simulink model "pokus07_video"  (R2023a)
settings: Solver=VariableStepAuto  StartTime=0.0  StopTime=10.0  RelTol=1e-3
undefined symbols (not defined in the file): c
libraries: Miscellaneous x840, Memory_Blocks_Lib x251, Decoders_Lib x10, simulink_extras x10, Counters_Lib x4, Bit_Multiplexers_Lib x1, Byte_Multiplexers_Lib x1
(part 4 of 5)

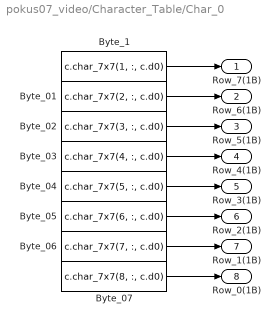
== system pokus07_video/Character_Table/Char_0 ==
  Byte_01 : Constant  Value=c.char_7x7(2, :, c.d0)  OutDataTypeStr=uint8
  Byte_02 : Constant  Value=c.char_7x7(3, :, c.d0)  OutDataTypeStr=uint8
  Byte_03 : Constant  Value=c.char_7x7(4, :, c.d0)  OutDataTypeStr=uint8
  Byte_04 : Constant  Value=c.char_7x7(5, :, c.d0)  OutDataTypeStr=uint8
  Byte_05 : Constant  Value=c.char_7x7(6, :, c.d0)  OutDataTypeStr=uint8
  Byte_06 : Constant  Value=c.char_7x7(7, :, c.d0)  OutDataTypeStr=uint8
  Byte_07 : Constant  Value=c.char_7x7(8, :, c.d0)  OutDataTypeStr=uint8
  Byte_1 : Constant  Value=c.char_7x7(1, :, c.d0)  OutDataTypeStr=uint8
  Row_7(1B) : Outport
  Row_6(1B) : Outport  Port=2
  Row_5(1B) : Outport  Port=3
  Row_4(1B) : Outport  Port=4
  Row_3(1B) : Outport  Port=5
  Row_2(1B) : Outport  Port=6
  Row_1(1B) : Outport  Port=7
  Row_0(1B) : Outport  Port=8
  wires:
  Byte_06/1 -> Row_1(1B)/1
  Byte_05/1 -> Row_2(1B)/1
  Byte_04/1 -> Row_3(1B)/1
  Byte_07/1 -> Row_0(1B)/1
  Byte_01/1 -> Row_6(1B)/1
  Byte_02/1 -> Row_5(1B)/1
  Byte_1/1 -> Row_7(1B)/1
  Byte_03/1 -> Row_4(1B)/1

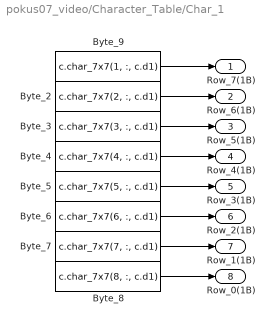
== system pokus07_video/Character_Table/Char_1 ==
  Byte_2 : Constant  Value=c.char_7x7(2, :, c.d1)  OutDataTypeStr=uint8
  Byte_3 : Constant  Value=c.char_7x7(3, :, c.d1)  OutDataTypeStr=uint8
  Byte_4 : Constant  Value=c.char_7x7(4, :, c.d1)  OutDataTypeStr=uint8
  Byte_5 : Constant  Value=c.char_7x7(5, :, c.d1)  OutDataTypeStr=uint8
  Byte_6 : Constant  Value=c.char_7x7(6, :, c.d1)  OutDataTypeStr=uint8
  Byte_7 : Constant  Value=c.char_7x7(7, :, c.d1)  OutDataTypeStr=uint8
  Byte_8 : Constant  Value=c.char_7x7(8, :, c.d1)  OutDataTypeStr=uint8
  Byte_9 : Constant  Value=c.char_7x7(1, :, c.d1)  OutDataTypeStr=uint8
  Row_7(1B) : Outport
  Row_6(1B) : Outport  Port=2
  Row_5(1B) : Outport  Port=3
  Row_4(1B) : Outport  Port=4
  Row_3(1B) : Outport  Port=5
  Row_2(1B) : Outport  Port=6
  Row_1(1B) : Outport  Port=7
  Row_0(1B) : Outport  Port=8
  wires:
  Byte_2/1 -> Row_6(1B)/1
  Byte_6/1 -> Row_2(1B)/1
  Byte_3/1 -> Row_5(1B)/1
  Byte_9/1 -> Row_7(1B)/1
  Byte_4/1 -> Row_4(1B)/1
  Byte_8/1 -> Row_0(1B)/1
  Byte_7/1 -> Row_1(1B)/1
  Byte_5/1 -> Row_3(1B)/1

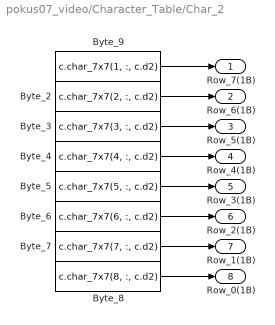
== system pokus07_video/Character_Table/Char_2 ==
  Byte_2 : Constant  Value=c.char_7x7(2, :, c.d2)  OutDataTypeStr=uint8
  Byte_3 : Constant  Value=c.char_7x7(3, :, c.d2)  OutDataTypeStr=uint8
  Byte_4 : Constant  Value=c.char_7x7(4, :, c.d2)  OutDataTypeStr=uint8
  Byte_5 : Constant  Value=c.char_7x7(5, :, c.d2)  OutDataTypeStr=uint8
  Byte_6 : Constant  Value=c.char_7x7(6, :, c.d2)  OutDataTypeStr=uint8
  Byte_7 : Constant  Value=c.char_7x7(7, :, c.d2)  OutDataTypeStr=uint8
  Byte_8 : Constant  Value=c.char_7x7(8, :, c.d2)  OutDataTypeStr=uint8
  Byte_9 : Constant  Value=c.char_7x7(1, :, c.d2)  OutDataTypeStr=uint8
  Row_7(1B) : Outport
  Row_6(1B) : Outport  Port=2
  Row_5(1B) : Outport  Port=3
  Row_4(1B) : Outport  Port=4
  Row_3(1B) : Outport  Port=5
  Row_2(1B) : Outport  Port=6
  Row_1(1B) : Outport  Port=7
  Row_0(1B) : Outport  Port=8
  wires:
  Byte_6/1 -> Row_2(1B)/1
  Byte_8/1 -> Row_0(1B)/1
  Byte_7/1 -> Row_1(1B)/1
  Byte_5/1 -> Row_3(1B)/1
  Byte_3/1 -> Row_5(1B)/1
  Byte_2/1 -> Row_6(1B)/1
  Byte_9/1 -> Row_7(1B)/1
  Byte_4/1 -> Row_4(1B)/1

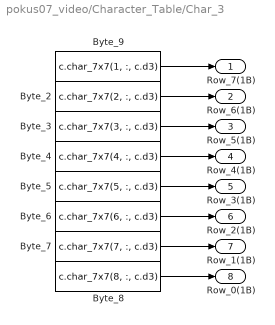
== system pokus07_video/Character_Table/Char_3 ==
  Byte_2 : Constant  Value=c.char_7x7(2, :, c.d3)  OutDataTypeStr=uint8
  Byte_3 : Constant  Value=c.char_7x7(3, :, c.d3)  OutDataTypeStr=uint8
  Byte_4 : Constant  Value=c.char_7x7(4, :, c.d3)  OutDataTypeStr=uint8
  Byte_5 : Constant  Value=c.char_7x7(5, :, c.d3)  OutDataTypeStr=uint8
  Byte_6 : Constant  Value=c.char_7x7(6, :, c.d3)  OutDataTypeStr=uint8
  Byte_7 : Constant  Value=c.char_7x7(7, :, c.d3)  OutDataTypeStr=uint8
  Byte_8 : Constant  Value=c.char_7x7(8, :, c.d3)  OutDataTypeStr=uint8
  Byte_9 : Constant  Value=c.char_7x7(1, :, c.d3)  OutDataTypeStr=uint8
  Row_7(1B) : Outport
  Row_6(1B) : Outport  Port=2
  Row_5(1B) : Outport  Port=3
  Row_4(1B) : Outport  Port=4
  Row_3(1B) : Outport  Port=5
  Row_2(1B) : Outport  Port=6
  Row_1(1B) : Outport  Port=7
  Row_0(1B) : Outport  Port=8
  wires:
  Byte_2/1 -> Row_6(1B)/1
  Byte_3/1 -> Row_5(1B)/1
  Byte_9/1 -> Row_7(1B)/1
  Byte_5/1 -> Row_3(1B)/1
  Byte_4/1 -> Row_4(1B)/1
  Byte_6/1 -> Row_2(1B)/1
  Byte_7/1 -> Row_1(1B)/1
  Byte_8/1 -> Row_0(1B)/1

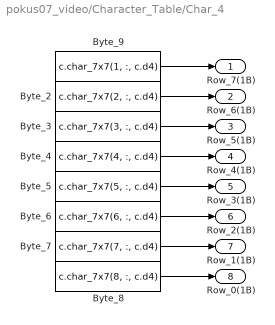
== system pokus07_video/Character_Table/Char_4 ==
  Byte_2 : Constant  Value=c.char_7x7(2, :, c.d4)  OutDataTypeStr=uint8
  Byte_3 : Constant  Value=c.char_7x7(3, :, c.d4)  OutDataTypeStr=uint8
  Byte_4 : Constant  Value=c.char_7x7(4, :, c.d4)  OutDataTypeStr=uint8
  Byte_5 : Constant  Value=c.char_7x7(5, :, c.d4)  OutDataTypeStr=uint8
  Byte_6 : Constant  Value=c.char_7x7(6, :, c.d4)  OutDataTypeStr=uint8
  Byte_7 : Constant  Value=c.char_7x7(7, :, c.d4)  OutDataTypeStr=uint8
  Byte_8 : Constant  Value=c.char_7x7(8, :, c.d4)  OutDataTypeStr=uint8
  Byte_9 : Constant  Value=c.char_7x7(1, :, c.d4)  OutDataTypeStr=uint8
  Row_7(1B) : Outport
  Row_6(1B) : Outport  Port=2
  Row_5(1B) : Outport  Port=3
  Row_4(1B) : Outport  Port=4
  Row_3(1B) : Outport  Port=5
  Row_2(1B) : Outport  Port=6
  Row_1(1B) : Outport  Port=7
  Row_0(1B) : Outport  Port=8
  wires:
  Byte_2/1 -> Row_6(1B)/1
  Byte_9/1 -> Row_7(1B)/1
  Byte_3/1 -> Row_5(1B)/1
  Byte_6/1 -> Row_2(1B)/1
  Byte_4/1 -> Row_4(1B)/1
  Byte_7/1 -> Row_1(1B)/1
  Byte_5/1 -> Row_3(1B)/1
  Byte_8/1 -> Row_0(1B)/1

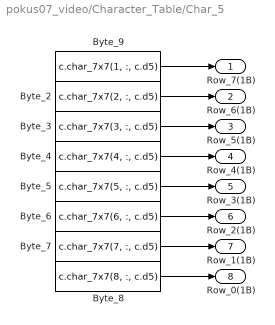
== system pokus07_video/Character_Table/Char_5 ==
  Byte_2 : Constant  Value=c.char_7x7(2, :, c.d5)  OutDataTypeStr=uint8
  Byte_3 : Constant  Value=c.char_7x7(3, :, c.d5)  OutDataTypeStr=uint8
  Byte_4 : Constant  Value=c.char_7x7(4, :, c.d5)  OutDataTypeStr=uint8
  Byte_5 : Constant  Value=c.char_7x7(5, :, c.d5)  OutDataTypeStr=uint8
  Byte_6 : Constant  Value=c.char_7x7(6, :, c.d5)  OutDataTypeStr=uint8
  Byte_7 : Constant  Value=c.char_7x7(7, :, c.d5)  OutDataTypeStr=uint8
  Byte_8 : Constant  Value=c.char_7x7(8, :, c.d5)  OutDataTypeStr=uint8
  Byte_9 : Constant  Value=c.char_7x7(1, :, c.d5)  OutDataTypeStr=uint8
  Row_7(1B) : Outport
  Row_6(1B) : Outport  Port=2
  Row_5(1B) : Outport  Port=3
  Row_4(1B) : Outport  Port=4
  Row_3(1B) : Outport  Port=5
  Row_2(1B) : Outport  Port=6
  Row_1(1B) : Outport  Port=7
  Row_0(1B) : Outport  Port=8
  wires:
  Byte_4/1 -> Row_4(1B)/1
  Byte_3/1 -> Row_5(1B)/1
  Byte_2/1 -> Row_6(1B)/1
  Byte_9/1 -> Row_7(1B)/1
  Byte_7/1 -> Row_1(1B)/1
  Byte_5/1 -> Row_3(1B)/1
  Byte_6/1 -> Row_2(1B)/1
  Byte_8/1 -> Row_0(1B)/1

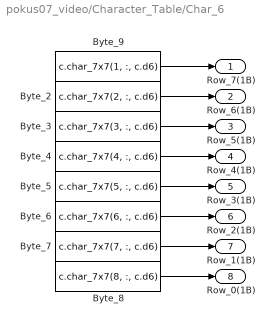
== system pokus07_video/Character_Table/Char_6 ==
  Byte_2 : Constant  Value=c.char_7x7(2, :, c.d6)  OutDataTypeStr=uint8
  Byte_3 : Constant  Value=c.char_7x7(3, :, c.d6)  OutDataTypeStr=uint8
  Byte_4 : Constant  Value=c.char_7x7(4, :, c.d6)  OutDataTypeStr=uint8
  Byte_5 : Constant  Value=c.char_7x7(5, :, c.d6)  OutDataTypeStr=uint8
  Byte_6 : Constant  Value=c.char_7x7(6, :, c.d6)  OutDataTypeStr=uint8
  Byte_7 : Constant  Value=c.char_7x7(7, :, c.d6)  OutDataTypeStr=uint8
  Byte_8 : Constant  Value=c.char_7x7(8, :, c.d6)  OutDataTypeStr=uint8
  Byte_9 : Constant  Value=c.char_7x7(1, :, c.d6)  OutDataTypeStr=uint8
  Row_7(1B) : Outport
  Row_6(1B) : Outport  Port=2
  Row_5(1B) : Outport  Port=3
  Row_4(1B) : Outport  Port=4
  Row_3(1B) : Outport  Port=5
  Row_2(1B) : Outport  Port=6
  Row_1(1B) : Outport  Port=7
  Row_0(1B) : Outport  Port=8
  wires:
  Byte_2/1 -> Row_6(1B)/1
  Byte_3/1 -> Row_5(1B)/1
  Byte_9/1 -> Row_7(1B)/1
  Byte_4/1 -> Row_4(1B)/1
  Byte_6/1 -> Row_2(1B)/1
  Byte_7/1 -> Row_1(1B)/1
  Byte_5/1 -> Row_3(1B)/1
  Byte_8/1 -> Row_0(1B)/1

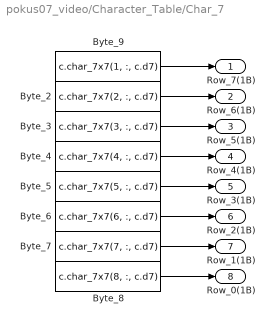
== system pokus07_video/Character_Table/Char_7 ==
  Byte_2 : Constant  Value=c.char_7x7(2, :, c.d7)  OutDataTypeStr=uint8
  Byte_3 : Constant  Value=c.char_7x7(3, :, c.d7)  OutDataTypeStr=uint8
  Byte_4 : Constant  Value=c.char_7x7(4, :, c.d7)  OutDataTypeStr=uint8
  Byte_5 : Constant  Value=c.char_7x7(5, :, c.d7)  OutDataTypeStr=uint8
  Byte_6 : Constant  Value=c.char_7x7(6, :, c.d7)  OutDataTypeStr=uint8
  Byte_7 : Constant  Value=c.char_7x7(7, :, c.d7)  OutDataTypeStr=uint8
  Byte_8 : Constant  Value=c.char_7x7(8, :, c.d7)  OutDataTypeStr=uint8
  Byte_9 : Constant  Value=c.char_7x7(1, :, c.d7)  OutDataTypeStr=uint8
  Row_7(1B) : Outport
  Row_6(1B) : Outport  Port=2
  Row_5(1B) : Outport  Port=3
  Row_4(1B) : Outport  Port=4
  Row_3(1B) : Outport  Port=5
  Row_2(1B) : Outport  Port=6
  Row_1(1B) : Outport  Port=7
  Row_0(1B) : Outport  Port=8
  wires:
  Byte_2/1 -> Row_6(1B)/1
  Byte_9/1 -> Row_7(1B)/1
  Byte_3/1 -> Row_5(1B)/1
  Byte_4/1 -> Row_4(1B)/1
  Byte_7/1 -> Row_1(1B)/1
  Byte_6/1 -> Row_2(1B)/1
  Byte_5/1 -> Row_3(1B)/1
  Byte_8/1 -> Row_0(1B)/1

== system pokus07_video/Character_Table/Char_8 ==
  Byte_2 : Constant  Value=c.char_7x7(2, :, c.d8)  OutDataTypeStr=uint8
  Byte_3 : Constant  Value=c.char_7x7(3, :, c.d8)  OutDataTypeStr=uint8
  Byte_4 : Constant  Value=c.char_7x7(4, :, c.d8)  OutDataTypeStr=uint8
  Byte_5 : Constant  Value=c.char_7x7(5, :, c.d8)  OutDataTypeStr=uint8
  Byte_6 : Constant  Value=c.char_7x7(6, :, c.d8)  OutDataTypeStr=uint8
  Byte_7 : Constant  Value=c.char_7x7(7, :, c.d8)  OutDataTypeStr=uint8
  Byte_8 : Constant  Value=c.char_7x7(8, :, c.d8)  OutDataTypeStr=uint8
  Byte_9 : Constant  Value=c.char_7x7(1, :, c.d8)  OutDataTypeStr=uint8
  Row_7(1B) : Outport
  Row_6(1B) : Outport  Port=2
  Row_5(1B) : Outport  Port=3
  Row_4(1B) : Outport  Port=4
  Row_3(1B) : Outport  Port=5
  Row_2(1B) : Outport  Port=6
  Row_1(1B) : Outport  Port=7
  Row_0(1B) : Outport  Port=8
  wires:
  Byte_5/1 -> Row_3(1B)/1
  Byte_7/1 -> Row_1(1B)/1
  Byte_8/1 -> Row_0(1B)/1
  Byte_4/1 -> Row_4(1B)/1
  Byte_2/1 -> Row_6(1B)/1
  Byte_3/1 -> Row_5(1B)/1
  Byte_6/1 -> Row_2(1B)/1
  Byte_9/1 -> Row_7(1B)/1

== system pokus07_video/Character_Table/Char_9 ==
  Byte_2 : Constant  Value=c.char_7x7(2, :, c.d9)  OutDataTypeStr=uint8
  Byte_3 : Constant  Value=c.char_7x7(3, :, c.d9)  OutDataTypeStr=uint8
  Byte_4 : Constant  Value=c.char_7x7(4, :, c.d9)  OutDataTypeStr=uint8
  Byte_5 : Constant  Value=c.char_7x7(5, :, c.d9)  OutDataTypeStr=uint8
  Byte_6 : Constant  Value=c.char_7x7(6, :, c.d9)  OutDataTypeStr=uint8
  Byte_7 : Constant  Value=c.char_7x7(7, :, c.d9)  OutDataTypeStr=uint8
  Byte_8 : Constant  Value=c.char_7x7(8, :, c.d9)  OutDataTypeStr=uint8
  Byte_9 : Constant  Value=c.char_7x7(1, :, c.d9)  OutDataTypeStr=uint8
  Row_7(1B) : Outport
  Row_6(1B) : Outport  Port=2
  Row_5(1B) : Outport  Port=3
  Row_4(1B) : Outport  Port=4
  Row_3(1B) : Outport  Port=5
  Row_2(1B) : Outport  Port=6
  Row_1(1B) : Outport  Port=7
  Row_0(1B) : Outport  Port=8
  wires:
  Byte_9/1 -> Row_7(1B)/1
  Byte_4/1 -> Row_4(1B)/1
  Byte_6/1 -> Row_2(1B)/1
  Byte_7/1 -> Row_1(1B)/1
  Byte_5/1 -> Row_3(1B)/1
  Byte_8/1 -> Row_0(1B)/1
  Byte_2/1 -> Row_6(1B)/1
  Byte_3/1 -> Row_5(1B)/1

== system pokus07_video/Character_Table/Char_A ==
  Byte_2 : Constant  Value=c.char_7x7(2, :, c.A)  OutDataTypeStr=uint8
  Byte_3 : Constant  Value=c.char_7x7(3, :, c.A)  OutDataTypeStr=uint8
  Byte_4 : Constant  Value=c.char_7x7(4, :, c.A)  OutDataTypeStr=uint8
  Byte_5 : Constant  Value=c.char_7x7(5, :, c.A)  OutDataTypeStr=uint8
  Byte_6 : Constant  Value=c.char_7x7(6, :, c.A)  OutDataTypeStr=uint8
  Byte_7 : Constant  Value=c.char_7x7(7, :, c.A)  OutDataTypeStr=uint8
  Byte_8 : Constant  Value=c.char_7x7(8, :, c.A)  OutDataTypeStr=uint8
  Byte_9 : Constant  Value=c.char_7x7(1, :, c.A)  OutDataTypeStr=uint8
  Row_7(1B) : Outport
  Row_6(1B) : Outport  Port=2
  Row_5(1B) : Outport  Port=3
  Row_4(1B) : Outport  Port=4
  Row_3(1B) : Outport  Port=5
  Row_2(1B) : Outport  Port=6
  Row_1(1B) : Outport  Port=7
  Row_0(1B) : Outport  Port=8
  wires:
  Byte_2/1 -> Row_6(1B)/1
  Byte_4/1 -> Row_4(1B)/1
  Byte_9/1 -> Row_7(1B)/1
  Byte_3/1 -> Row_5(1B)/1
  Byte_6/1 -> Row_2(1B)/1
  Byte_7/1 -> Row_1(1B)/1
  Byte_5/1 -> Row_3(1B)/1
  Byte_8/1 -> Row_0(1B)/1

== system pokus07_video/Character_Table/Char_ASTERISK ==
  Byte_2 : Constant  Value=c.char_7x7(2, :, c.ASTERISK)  OutDataTypeStr=uint8
  Byte_3 : Constant  Value=c.char_7x7(3, :, c.ASTERISK)  OutDataTypeStr=uint8
  Byte_4 : Constant  Value=c.char_7x7(4, :, c.ASTERISK)  OutDataTypeStr=uint8
  Byte_5 : Constant  Value=c.char_7x7(5, :, c.ASTERISK)  OutDataTypeStr=uint8
  Byte_6 : Constant  Value=c.char_7x7(6, :, c.ASTERISK)  OutDataTypeStr=uint8
  Byte_7 : Constant  Value=c.char_7x7(7, :, c.ASTERISK)  OutDataTypeStr=uint8
  Byte_8 : Constant  Value=c.char_7x7(8, :, c.ASTERISK)  OutDataTypeStr=uint8
  Byte_9 : Constant  Value=c.char_7x7(1, :, c.ASTERISK)  OutDataTypeStr=uint8
  Row_7(1B) : Outport
  Row_6(1B) : Outport  Port=2
  Row_5(1B) : Outport  Port=3
  Row_4(1B) : Outport  Port=4
  Row_3(1B) : Outport  Port=5
  Row_2(1B) : Outport  Port=6
  Row_1(1B) : Outport  Port=7
  Row_0(1B) : Outport  Port=8
  wires:
  Byte_3/1 -> Row_5(1B)/1
  Byte_9/1 -> Row_7(1B)/1
  Byte_7/1 -> Row_1(1B)/1
  Byte_4/1 -> Row_4(1B)/1
  Byte_8/1 -> Row_0(1B)/1
  Byte_2/1 -> Row_6(1B)/1
  Byte_5/1 -> Row_3(1B)/1
  Byte_6/1 -> Row_2(1B)/1

== system pokus07_video/Character_Table/Char_B ==
  Byte_2 : Constant  Value=c.char_7x7(2, :, c.B)  OutDataTypeStr=uint8
  Byte_3 : Constant  Value=c.char_7x7(3, :, c.B)  OutDataTypeStr=uint8
  Byte_4 : Constant  Value=c.char_7x7(4, :, c.B)  OutDataTypeStr=uint8
  Byte_5 : Constant  Value=c.char_7x7(5, :, c.B)  OutDataTypeStr=uint8
  Byte_6 : Constant  Value=c.char_7x7(6, :, c.B)  OutDataTypeStr=uint8
  Byte_7 : Constant  Value=c.char_7x7(7, :, c.B)  OutDataTypeStr=uint8
  Byte_8 : Constant  Value=c.char_7x7(8, :, c.B)  OutDataTypeStr=uint8
  Byte_9 : Constant  Value=c.char_7x7(1, :, c.B)  OutDataTypeStr=uint8
  Row_7(1B) : Outport
  Row_6(1B) : Outport  Port=2
  Row_5(1B) : Outport  Port=3
  Row_4(1B) : Outport  Port=4
  Row_3(1B) : Outport  Port=5
  Row_2(1B) : Outport  Port=6
  Row_1(1B) : Outport  Port=7
  Row_0(1B) : Outport  Port=8
  wires:
  Byte_2/1 -> Row_6(1B)/1
  Byte_7/1 -> Row_1(1B)/1
  Byte_3/1 -> Row_5(1B)/1
  Byte_4/1 -> Row_4(1B)/1
  Byte_9/1 -> Row_7(1B)/1
  Byte_6/1 -> Row_2(1B)/1
  Byte_5/1 -> Row_3(1B)/1
  Byte_8/1 -> Row_0(1B)/1

== system pokus07_video/Character_Table/Char_BACKSLASH ==
  Byte_2 : Constant  Value=c.char_7x7(2, :, c.BACKSLASH)  OutDataTypeStr=uint8
  Byte_3 : Constant  Value=c.char_7x7(3, :, c.BACKSLASH)  OutDataTypeStr=uint8
  Byte_4 : Constant  Value=c.char_7x7(4, :, c.BACKSLASH)  OutDataTypeStr=uint8
  Byte_5 : Constant  Value=c.char_7x7(5, :, c.BACKSLASH)  OutDataTypeStr=uint8
  Byte_6 : Constant  Value=c.char_7x7(6, :, c.BACKSLASH)  OutDataTypeStr=uint8
  Byte_7 : Constant  Value=c.char_7x7(7, :, c.BACKSLASH)  OutDataTypeStr=uint8
  Byte_8 : Constant  Value=c.char_7x7(8, :, c.BACKSLASH)  OutDataTypeStr=uint8
  Byte_9 : Constant  Value=c.char_7x7(1, :, c.BACKSLASH)  OutDataTypeStr=uint8
  Row_7(1B) : Outport
  Row_6(1B) : Outport  Port=2
  Row_5(1B) : Outport  Port=3
  Row_4(1B) : Outport  Port=4
  Row_3(1B) : Outport  Port=5
  Row_2(1B) : Outport  Port=6
  Row_1(1B) : Outport  Port=7
  Row_0(1B) : Outport  Port=8
  wires:
  Byte_3/1 -> Row_5(1B)/1
  Byte_9/1 -> Row_7(1B)/1
  Byte_7/1 -> Row_1(1B)/1
  Byte_4/1 -> Row_4(1B)/1
  Byte_8/1 -> Row_0(1B)/1
  Byte_2/1 -> Row_6(1B)/1
  Byte_5/1 -> Row_3(1B)/1
  Byte_6/1 -> Row_2(1B)/1

== system pokus07_video/Character_Table/Char_C ==
  Byte_2 : Constant  Value=c.char_7x7(2, :, c.C)  OutDataTypeStr=uint8
  Byte_3 : Constant  Value=c.char_7x7(3, :, c.C)  OutDataTypeStr=uint8
  Byte_4 : Constant  Value=c.char_7x7(4, :, c.C)  OutDataTypeStr=uint8
  Byte_5 : Constant  Value=c.char_7x7(5, :, c.C)  OutDataTypeStr=uint8
  Byte_6 : Constant  Value=c.char_7x7(6, :, c.C)  OutDataTypeStr=uint8
  Byte_7 : Constant  Value=c.char_7x7(7, :, c.C)  OutDataTypeStr=uint8
  Byte_8 : Constant  Value=c.char_7x7(8, :, c.C)  OutDataTypeStr=uint8
  Byte_9 : Constant  Value=c.char_7x7(1, :, c.C)  OutDataTypeStr=uint8
  Row_7(1B) : Outport
  Row_6(1B) : Outport  Port=2
  Row_5(1B) : Outport  Port=3
  Row_4(1B) : Outport  Port=4
  Row_3(1B) : Outport  Port=5
  Row_2(1B) : Outport  Port=6
  Row_1(1B) : Outport  Port=7
  Row_0(1B) : Outport  Port=8
  wires:
  Byte_9/1 -> Row_7(1B)/1
  Byte_2/1 -> Row_6(1B)/1
  Byte_3/1 -> Row_5(1B)/1
  Byte_4/1 -> Row_4(1B)/1
  Byte_5/1 -> Row_3(1B)/1
  Byte_6/1 -> Row_2(1B)/1
  Byte_7/1 -> Row_1(1B)/1
  Byte_8/1 -> Row_0(1B)/1

== system pokus07_video/Character_Table/Char_COLON ==
  Byte_2 : Constant  Value=c.char_7x7(2, :, c.COLON)  OutDataTypeStr=uint8
  Byte_3 : Constant  Value=c.char_7x7(3, :, c.COLON)  OutDataTypeStr=uint8
  Byte_4 : Constant  Value=c.char_7x7(4, :, c.COLON)  OutDataTypeStr=uint8
  Byte_5 : Constant  Value=c.char_7x7(5, :, c.COLON)  OutDataTypeStr=uint8
  Byte_6 : Constant  Value=c.char_7x7(6, :, c.COLON)  OutDataTypeStr=uint8
  Byte_7 : Constant  Value=c.char_7x7(7, :, c.COLON)  OutDataTypeStr=uint8
  Byte_8 : Constant  Value=c.char_7x7(8, :, c.COLON)  OutDataTypeStr=uint8
  Byte_9 : Constant  Value=c.char_7x7(1, :, c.COLON)  OutDataTypeStr=uint8
  Row_7(1B) : Outport
  Row_6(1B) : Outport  Port=2
  Row_5(1B) : Outport  Port=3
  Row_4(1B) : Outport  Port=4
  Row_3(1B) : Outport  Port=5
  Row_2(1B) : Outport  Port=6
  Row_1(1B) : Outport  Port=7
  Row_0(1B) : Outport  Port=8
  wires:
  Byte_3/1 -> Row_5(1B)/1
  Byte_9/1 -> Row_7(1B)/1
  Byte_7/1 -> Row_1(1B)/1
  Byte_4/1 -> Row_4(1B)/1
  Byte_8/1 -> Row_0(1B)/1
  Byte_2/1 -> Row_6(1B)/1
  Byte_5/1 -> Row_3(1B)/1
  Byte_6/1 -> Row_2(1B)/1

== system pokus07_video/Character_Table/Char_COMMA ==
  Byte_2 : Constant  Value=c.char_7x7(2, :, c.COMMA)  OutDataTypeStr=uint8
  Byte_3 : Constant  Value=c.char_7x7(3, :, c.COMMA)  OutDataTypeStr=uint8
  Byte_4 : Constant  Value=c.char_7x7(4, :, c.COMMA)  OutDataTypeStr=uint8
  Byte_5 : Constant  Value=c.char_7x7(5, :, c.COMMA)  OutDataTypeStr=uint8
  Byte_6 : Constant  Value=c.char_7x7(6, :, c.COMMA)  OutDataTypeStr=uint8
  Byte_7 : Constant  Value=c.char_7x7(7, :, c.COMMA)  OutDataTypeStr=uint8
  Byte_8 : Constant  Value=c.char_7x7(8, :, c.COMMA)  OutDataTypeStr=uint8
  Byte_9 : Constant  Value=c.char_7x7(1, :, c.COMMA)  OutDataTypeStr=uint8
  Row_7(1B) : Outport
  Row_6(1B) : Outport  Port=2
  Row_5(1B) : Outport  Port=3
  Row_4(1B) : Outport  Port=4
  Row_3(1B) : Outport  Port=5
  Row_2(1B) : Outport  Port=6
  Row_1(1B) : Outport  Port=7
  Row_0(1B) : Outport  Port=8
  wires:
  Byte_3/1 -> Row_5(1B)/1
  Byte_9/1 -> Row_7(1B)/1
  Byte_7/1 -> Row_1(1B)/1
  Byte_4/1 -> Row_4(1B)/1
  Byte_8/1 -> Row_0(1B)/1
  Byte_2/1 -> Row_6(1B)/1
  Byte_5/1 -> Row_3(1B)/1
  Byte_6/1 -> Row_2(1B)/1

== system pokus07_video/Character_Table/Char_D ==
  Byte_2 : Constant  Value=c.char_7x7(2, :, c.D)  OutDataTypeStr=uint8
  Byte_3 : Constant  Value=c.char_7x7(3, :, c.D)  OutDataTypeStr=uint8
  Byte_4 : Constant  Value=c.char_7x7(4, :, c.D)  OutDataTypeStr=uint8
  Byte_5 : Constant  Value=c.char_7x7(5, :, c.D)  OutDataTypeStr=uint8
  Byte_6 : Constant  Value=c.char_7x7(6, :, c.D)  OutDataTypeStr=uint8
  Byte_7 : Constant  Value=c.char_7x7(7, :, c.D)  OutDataTypeStr=uint8
  Byte_8 : Constant  Value=c.char_7x7(8, :, c.D)  OutDataTypeStr=uint8
  Byte_9 : Constant  Value=c.char_7x7(1, :, c.D)  OutDataTypeStr=uint8
  Row_7(1B) : Outport
  Row_6(1B) : Outport  Port=2
  Row_5(1B) : Outport  Port=3
  Row_4(1B) : Outport  Port=4
  Row_3(1B) : Outport  Port=5
  Row_2(1B) : Outport  Port=6
  Row_1(1B) : Outport  Port=7
  Row_0(1B) : Outport  Port=8
  wires:
  Byte_2/1 -> Row_6(1B)/1
  Byte_3/1 -> Row_5(1B)/1
  Byte_9/1 -> Row_7(1B)/1
  Byte_4/1 -> Row_4(1B)/1
  Byte_6/1 -> Row_2(1B)/1
  Byte_7/1 -> Row_1(1B)/1
  Byte_5/1 -> Row_3(1B)/1
  Byte_8/1 -> Row_0(1B)/1

== system pokus07_video/Character_Table/Char_DOT ==
  Byte_2 : Constant  Value=c.char_7x7(2, :, c.DOT)  OutDataTypeStr=uint8
  Byte_3 : Constant  Value=c.char_7x7(3, :, c.DOT)  OutDataTypeStr=uint8
  Byte_4 : Constant  Value=c.char_7x7(4, :, c.DOT)  OutDataTypeStr=uint8
  Byte_5 : Constant  Value=c.char_7x7(5, :, c.DOT)  OutDataTypeStr=uint8
  Byte_6 : Constant  Value=c.char_7x7(6, :, c.DOT)  OutDataTypeStr=uint8
  Byte_7 : Constant  Value=c.char_7x7(7, :, c.DOT)  OutDataTypeStr=uint8
  Byte_8 : Constant  Value=c.char_7x7(8, :, c.DOT)  OutDataTypeStr=uint8
  Byte_9 : Constant  Value=c.char_7x7(1, :, c.DOT)  OutDataTypeStr=uint8
  Row_7(1B) : Outport
  Row_6(1B) : Outport  Port=2
  Row_5(1B) : Outport  Port=3
  Row_4(1B) : Outport  Port=4
  Row_3(1B) : Outport  Port=5
  Row_2(1B) : Outport  Port=6
  Row_1(1B) : Outport  Port=7
  Row_0(1B) : Outport  Port=8
  wires:
  Byte_3/1 -> Row_5(1B)/1
  Byte_9/1 -> Row_7(1B)/1
  Byte_7/1 -> Row_1(1B)/1
  Byte_4/1 -> Row_4(1B)/1
  Byte_8/1 -> Row_0(1B)/1
  Byte_2/1 -> Row_6(1B)/1
  Byte_5/1 -> Row_3(1B)/1
  Byte_6/1 -> Row_2(1B)/1

== system pokus07_video/Character_Table/Char_E ==
  Byte_2 : Constant  Value=c.char_7x7(2, :, c.E)  OutDataTypeStr=uint8
  Byte_3 : Constant  Value=c.char_7x7(3, :, c.E)  OutDataTypeStr=uint8
  Byte_4 : Constant  Value=c.char_7x7(4, :, c.E)  OutDataTypeStr=uint8
  Byte_5 : Constant  Value=c.char_7x7(5, :, c.E)  OutDataTypeStr=uint8
  Byte_6 : Constant  Value=c.char_7x7(6, :, c.E)  OutDataTypeStr=uint8
  Byte_7 : Constant  Value=c.char_7x7(7, :, c.E)  OutDataTypeStr=uint8
  Byte_8 : Constant  Value=c.char_7x7(8, :, c.E)  OutDataTypeStr=uint8
  Byte_9 : Constant  Value=c.char_7x7(1, :, c.E)  OutDataTypeStr=uint8
  Row_7(1B) : Outport
  Row_6(1B) : Outport  Port=2
  Row_5(1B) : Outport  Port=3
  Row_4(1B) : Outport  Port=4
  Row_3(1B) : Outport  Port=5
  Row_2(1B) : Outport  Port=6
  Row_1(1B) : Outport  Port=7
  Row_0(1B) : Outport  Port=8
  wires:
  Byte_2/1 -> Row_6(1B)/1
  Byte_9/1 -> Row_7(1B)/1
  Byte_6/1 -> Row_2(1B)/1
  Byte_3/1 -> Row_5(1B)/1
  Byte_7/1 -> Row_1(1B)/1
  Byte_5/1 -> Row_3(1B)/1
  Byte_4/1 -> Row_4(1B)/1
  Byte_8/1 -> Row_0(1B)/1

== system pokus07_video/Character_Table/Char_EQUAL ==
  Byte_2 : Constant  Value=c.char_7x7(2, :, c.EQUALS)  OutDataTypeStr=uint8
  Byte_3 : Constant  Value=c.char_7x7(3, :, c.EQUALS)  OutDataTypeStr=uint8
  Byte_4 : Constant  Value=c.char_7x7(4, :, c.EQUALS)  OutDataTypeStr=uint8
  Byte_5 : Constant  Value=c.char_7x7(5, :, c.EQUALS)  OutDataTypeStr=uint8
  Byte_6 : Constant  Value=c.char_7x7(6, :, c.EQUALS)  OutDataTypeStr=uint8
  Byte_7 : Constant  Value=c.char_7x7(7, :, c.EQUALS)  OutDataTypeStr=uint8
  Byte_8 : Constant  Value=c.char_7x7(8, :, c.EQUALS)  OutDataTypeStr=uint8
  Byte_9 : Constant  Value=c.char_7x7(1, :, c.EQUALS)  OutDataTypeStr=uint8
  Row_7(1B) : Outport
  Row_6(1B) : Outport  Port=2
  Row_5(1B) : Outport  Port=3
  Row_4(1B) : Outport  Port=4
  Row_3(1B) : Outport  Port=5
  Row_2(1B) : Outport  Port=6
  Row_1(1B) : Outport  Port=7
  Row_0(1B) : Outport  Port=8
  wires:
  Byte_3/1 -> Row_5(1B)/1
  Byte_9/1 -> Row_7(1B)/1
  Byte_7/1 -> Row_1(1B)/1
  Byte_4/1 -> Row_4(1B)/1
  Byte_8/1 -> Row_0(1B)/1
  Byte_2/1 -> Row_6(1B)/1
  Byte_5/1 -> Row_3(1B)/1
  Byte_6/1 -> Row_2(1B)/1

== system pokus07_video/Character_Table/Char_EXCLAMATION_MARK ==
  Byte_2 : Constant  Value=c.char_7x7(2, :, c.EXCLAMATION_MARK)  OutDataTypeStr=uint8
  Byte_3 : Constant  Value=c.char_7x7(3, :, c.EXCLAMATION_MARK)  OutDataTypeStr=uint8
  Byte_4 : Constant  Value=c.char_7x7(4, :, c.EXCLAMATION_MARK)  OutDataTypeStr=uint8
  Byte_5 : Constant  Value=c.char_7x7(5, :, c.EXCLAMATION_MARK)  OutDataTypeStr=uint8
  Byte_6 : Constant  Value=c.char_7x7(6, :, c.EXCLAMATION_MARK)  OutDataTypeStr=uint8
  Byte_7 : Constant  Value=c.char_7x7(7, :, c.EXCLAMATION_MARK)  OutDataTypeStr=uint8
  Byte_8 : Constant  Value=c.char_7x7(8, :, c.EXCLAMATION_MARK)  OutDataTypeStr=uint8
  Byte_9 : Constant  Value=c.char_7x7(1, :, c.EXCLAMATION_MARK)  OutDataTypeStr=uint8
  Row_7(1B) : Outport
  Row_6(1B) : Outport  Port=2
  Row_5(1B) : Outport  Port=3
  Row_4(1B) : Outport  Port=4
  Row_3(1B) : Outport  Port=5
  Row_2(1B) : Outport  Port=6
  Row_1(1B) : Outport  Port=7
  Row_0(1B) : Outport  Port=8
  wires:
  Byte_3/1 -> Row_5(1B)/1
  Byte_9/1 -> Row_7(1B)/1
  Byte_7/1 -> Row_1(1B)/1
  Byte_4/1 -> Row_4(1B)/1
  Byte_8/1 -> Row_0(1B)/1
  Byte_2/1 -> Row_6(1B)/1
  Byte_5/1 -> Row_3(1B)/1
  Byte_6/1 -> Row_2(1B)/1

== system pokus07_video/Character_Table/Char_EXCLAMATION_MARK1 ==
  Byte_2 : Constant  Value=c.char_7x7(2, :, c.EXCLAMATION_MARK)  OutDataTypeStr=uint8
  Byte_3 : Constant  Value=c.char_7x7(3, :, c.EXCLAMATION_MARK)  OutDataTypeStr=uint8
  Byte_4 : Constant  Value=c.char_7x7(4, :, c.EXCLAMATION_MARK)  OutDataTypeStr=uint8
  Byte_5 : Constant  Value=c.char_7x7(5, :, c.EXCLAMATION_MARK)  OutDataTypeStr=uint8
  Byte_6 : Constant  Value=c.char_7x7(6, :, c.EXCLAMATION_MARK)  OutDataTypeStr=uint8
  Byte_7 : Constant  Value=c.char_7x7(7, :, c.EXCLAMATION_MARK)  OutDataTypeStr=uint8
  Byte_8 : Constant  Value=c.char_7x7(8, :, c.EXCLAMATION_MARK)  OutDataTypeStr=uint8
  Byte_9 : Constant  Value=c.char_7x7(1, :, c.EXCLAMATION_MARK)  OutDataTypeStr=uint8
  Row_7(1B) : Outport
  Row_6(1B) : Outport  Port=2
  Row_5(1B) : Outport  Port=3
  Row_4(1B) : Outport  Port=4
  Row_3(1B) : Outport  Port=5
  Row_2(1B) : Outport  Port=6
  Row_1(1B) : Outport  Port=7
  Row_0(1B) : Outport  Port=8
  wires:
  Byte_3/1 -> Row_5(1B)/1
  Byte_9/1 -> Row_7(1B)/1
  Byte_7/1 -> Row_1(1B)/1
  Byte_4/1 -> Row_4(1B)/1
  Byte_8/1 -> Row_0(1B)/1
  Byte_2/1 -> Row_6(1B)/1
  Byte_5/1 -> Row_3(1B)/1
  Byte_6/1 -> Row_2(1B)/1

== system pokus07_video/Character_Table/Char_EXCLAMATION_MARK10 ==
  Byte_2 : Constant  Value=c.char_7x7(2, :, c.EXCLAMATION_MARK)  OutDataTypeStr=uint8
  Byte_3 : Constant  Value=c.char_7x7(3, :, c.EXCLAMATION_MARK)  OutDataTypeStr=uint8
  Byte_4 : Constant  Value=c.char_7x7(4, :, c.EXCLAMATION_MARK)  OutDataTypeStr=uint8
  Byte_5 : Constant  Value=c.char_7x7(5, :, c.EXCLAMATION_MARK)  OutDataTypeStr=uint8
  Byte_6 : Constant  Value=c.char_7x7(6, :, c.EXCLAMATION_MARK)  OutDataTypeStr=uint8
  Byte_7 : Constant  Value=c.char_7x7(7, :, c.EXCLAMATION_MARK)  OutDataTypeStr=uint8
  Byte_8 : Constant  Value=c.char_7x7(8, :, c.EXCLAMATION_MARK)  OutDataTypeStr=uint8
  Byte_9 : Constant  Value=c.char_7x7(1, :, c.EXCLAMATION_MARK)  OutDataTypeStr=uint8
  Row_7(1B) : Outport
  Row_6(1B) : Outport  Port=2
  Row_5(1B) : Outport  Port=3
  Row_4(1B) : Outport  Port=4
  Row_3(1B) : Outport  Port=5
  Row_2(1B) : Outport  Port=6
  Row_1(1B) : Outport  Port=7
  Row_0(1B) : Outport  Port=8
  wires:
  Byte_2/1 -> Row_6(1B)/1
  Byte_9/1 -> Row_7(1B)/1
  Byte_3/1 -> Row_5(1B)/1
  Byte_4/1 -> Row_4(1B)/1
  Byte_5/1 -> Row_3(1B)/1
  Byte_6/1 -> Row_2(1B)/1
  Byte_7/1 -> Row_1(1B)/1
  Byte_8/1 -> Row_0(1B)/1

== system pokus07_video/Character_Table/Char_EXCLAMATION_MARK11 ==
  Byte_2 : Constant  Value=c.char_7x7(2, :, c.EXCLAMATION_MARK)  OutDataTypeStr=uint8
  Byte_3 : Constant  Value=c.char_7x7(3, :, c.EXCLAMATION_MARK)  OutDataTypeStr=uint8
  Byte_4 : Constant  Value=c.char_7x7(4, :, c.EXCLAMATION_MARK)  OutDataTypeStr=uint8
  Byte_5 : Constant  Value=c.char_7x7(5, :, c.EXCLAMATION_MARK)  OutDataTypeStr=uint8
  Byte_6 : Constant  Value=c.char_7x7(6, :, c.EXCLAMATION_MARK)  OutDataTypeStr=uint8
  Byte_7 : Constant  Value=c.char_7x7(7, :, c.EXCLAMATION_MARK)  OutDataTypeStr=uint8
  Byte_8 : Constant  Value=c.char_7x7(8, :, c.EXCLAMATION_MARK)  OutDataTypeStr=uint8
  Byte_9 : Constant  Value=c.char_7x7(1, :, c.EXCLAMATION_MARK)  OutDataTypeStr=uint8
  Row_7(1B) : Outport
  Row_6(1B) : Outport  Port=2
  Row_5(1B) : Outport  Port=3
  Row_4(1B) : Outport  Port=4
  Row_3(1B) : Outport  Port=5
  Row_2(1B) : Outport  Port=6
  Row_1(1B) : Outport  Port=7
  Row_0(1B) : Outport  Port=8
  wires:
  Byte_3/1 -> Row_5(1B)/1
  Byte_9/1 -> Row_7(1B)/1
  Byte_7/1 -> Row_1(1B)/1
  Byte_4/1 -> Row_4(1B)/1
  Byte_8/1 -> Row_0(1B)/1
  Byte_2/1 -> Row_6(1B)/1
  Byte_5/1 -> Row_3(1B)/1
  Byte_6/1 -> Row_2(1B)/1

== system pokus07_video/Character_Table/Char_EXCLAMATION_MARK2 ==
  Byte_2 : Constant  Value=c.char_7x7(2, :, c.EXCLAMATION_MARK)  OutDataTypeStr=uint8
  Byte_3 : Constant  Value=c.char_7x7(3, :, c.EXCLAMATION_MARK)  OutDataTypeStr=uint8
  Byte_4 : Constant  Value=c.char_7x7(4, :, c.EXCLAMATION_MARK)  OutDataTypeStr=uint8
  Byte_5 : Constant  Value=c.char_7x7(5, :, c.EXCLAMATION_MARK)  OutDataTypeStr=uint8
  Byte_6 : Constant  Value=c.char_7x7(6, :, c.EXCLAMATION_MARK)  OutDataTypeStr=uint8
  Byte_7 : Constant  Value=c.char_7x7(7, :, c.EXCLAMATION_MARK)  OutDataTypeStr=uint8
  Byte_8 : Constant  Value=c.char_7x7(8, :, c.EXCLAMATION_MARK)  OutDataTypeStr=uint8
  Byte_9 : Constant  Value=c.char_7x7(1, :, c.EXCLAMATION_MARK)  OutDataTypeStr=uint8
  Row_7(1B) : Outport
  Row_6(1B) : Outport  Port=2
  Row_5(1B) : Outport  Port=3
  Row_4(1B) : Outport  Port=4
  Row_3(1B) : Outport  Port=5
  Row_2(1B) : Outport  Port=6
  Row_1(1B) : Outport  Port=7
  Row_0(1B) : Outport  Port=8
  wires:
  Byte_3/1 -> Row_5(1B)/1
  Byte_9/1 -> Row_7(1B)/1
  Byte_7/1 -> Row_1(1B)/1
  Byte_4/1 -> Row_4(1B)/1
  Byte_8/1 -> Row_0(1B)/1
  Byte_2/1 -> Row_6(1B)/1
  Byte_5/1 -> Row_3(1B)/1
  Byte_6/1 -> Row_2(1B)/1

== system pokus07_video/Character_Table/Char_EXCLAMATION_MARK3 ==
  Byte_2 : Constant  Value=c.char_7x7(2, :, c.EXCLAMATION_MARK)  OutDataTypeStr=uint8
  Byte_3 : Constant  Value=c.char_7x7(3, :, c.EXCLAMATION_MARK)  OutDataTypeStr=uint8
  Byte_4 : Constant  Value=c.char_7x7(4, :, c.EXCLAMATION_MARK)  OutDataTypeStr=uint8
  Byte_5 : Constant  Value=c.char_7x7(5, :, c.EXCLAMATION_MARK)  OutDataTypeStr=uint8
  Byte_6 : Constant  Value=c.char_7x7(6, :, c.EXCLAMATION_MARK)  OutDataTypeStr=uint8
  Byte_7 : Constant  Value=c.char_7x7(7, :, c.EXCLAMATION_MARK)  OutDataTypeStr=uint8
  Byte_8 : Constant  Value=c.char_7x7(8, :, c.EXCLAMATION_MARK)  OutDataTypeStr=uint8
  Byte_9 : Constant  Value=c.char_7x7(1, :, c.EXCLAMATION_MARK)  OutDataTypeStr=uint8
  Row_7(1B) : Outport
  Row_6(1B) : Outport  Port=2
  Row_5(1B) : Outport  Port=3
  Row_4(1B) : Outport  Port=4
  Row_3(1B) : Outport  Port=5
  Row_2(1B) : Outport  Port=6
  Row_1(1B) : Outport  Port=7
  Row_0(1B) : Outport  Port=8
  wires:
  Byte_3/1 -> Row_5(1B)/1
  Byte_9/1 -> Row_7(1B)/1
  Byte_7/1 -> Row_1(1B)/1
  Byte_4/1 -> Row_4(1B)/1
  Byte_8/1 -> Row_0(1B)/1
  Byte_2/1 -> Row_6(1B)/1
  Byte_5/1 -> Row_3(1B)/1
  Byte_6/1 -> Row_2(1B)/1

== system pokus07_video/Character_Table/Char_EXCLAMATION_MARK4 ==
  Byte_2 : Constant  Value=c.char_7x7(2, :, c.EXCLAMATION_MARK)  OutDataTypeStr=uint8
  Byte_3 : Constant  Value=c.char_7x7(3, :, c.EXCLAMATION_MARK)  OutDataTypeStr=uint8
  Byte_4 : Constant  Value=c.char_7x7(4, :, c.EXCLAMATION_MARK)  OutDataTypeStr=uint8
  Byte_5 : Constant  Value=c.char_7x7(5, :, c.EXCLAMATION_MARK)  OutDataTypeStr=uint8
  Byte_6 : Constant  Value=c.char_7x7(6, :, c.EXCLAMATION_MARK)  OutDataTypeStr=uint8
  Byte_7 : Constant  Value=c.char_7x7(7, :, c.EXCLAMATION_MARK)  OutDataTypeStr=uint8
  Byte_8 : Constant  Value=c.char_7x7(8, :, c.EXCLAMATION_MARK)  OutDataTypeStr=uint8
  Byte_9 : Constant  Value=c.char_7x7(1, :, c.EXCLAMATION_MARK)  OutDataTypeStr=uint8
  Row_7(1B) : Outport
  Row_6(1B) : Outport  Port=2
  Row_5(1B) : Outport  Port=3
  Row_4(1B) : Outport  Port=4
  Row_3(1B) : Outport  Port=5
  Row_2(1B) : Outport  Port=6
  Row_1(1B) : Outport  Port=7
  Row_0(1B) : Outport  Port=8
  wires:
  Byte_3/1 -> Row_5(1B)/1
  Byte_9/1 -> Row_7(1B)/1
  Byte_7/1 -> Row_1(1B)/1
  Byte_4/1 -> Row_4(1B)/1
  Byte_8/1 -> Row_0(1B)/1
  Byte_2/1 -> Row_6(1B)/1
  Byte_5/1 -> Row_3(1B)/1
  Byte_6/1 -> Row_2(1B)/1

== system pokus07_video/Character_Table/Char_EXCLAMATION_MARK5 ==
  Byte_2 : Constant  Value=c.char_7x7(2, :, c.EXCLAMATION_MARK)  OutDataTypeStr=uint8
  Byte_3 : Constant  Value=c.char_7x7(3, :, c.EXCLAMATION_MARK)  OutDataTypeStr=uint8
  Byte_4 : Constant  Value=c.char_7x7(4, :, c.EXCLAMATION_MARK)  OutDataTypeStr=uint8
  Byte_5 : Constant  Value=c.char_7x7(5, :, c.EXCLAMATION_MARK)  OutDataTypeStr=uint8
  Byte_6 : Constant  Value=c.char_7x7(6, :, c.EXCLAMATION_MARK)  OutDataTypeStr=uint8
  Byte_7 : Constant  Value=c.char_7x7(7, :, c.EXCLAMATION_MARK)  OutDataTypeStr=uint8
  Byte_8 : Constant  Value=c.char_7x7(8, :, c.EXCLAMATION_MARK)  OutDataTypeStr=uint8
  Byte_9 : Constant  Value=c.char_7x7(1, :, c.EXCLAMATION_MARK)  OutDataTypeStr=uint8
  Row_7(1B) : Outport
  Row_6(1B) : Outport  Port=2
  Row_5(1B) : Outport  Port=3
  Row_4(1B) : Outport  Port=4
  Row_3(1B) : Outport  Port=5
  Row_2(1B) : Outport  Port=6
  Row_1(1B) : Outport  Port=7
  Row_0(1B) : Outport  Port=8
  wires:
  Byte_3/1 -> Row_5(1B)/1
  Byte_9/1 -> Row_7(1B)/1
  Byte_7/1 -> Row_1(1B)/1
  Byte_4/1 -> Row_4(1B)/1
  Byte_8/1 -> Row_0(1B)/1
  Byte_2/1 -> Row_6(1B)/1
  Byte_5/1 -> Row_3(1B)/1
  Byte_6/1 -> Row_2(1B)/1

== system pokus07_video/Character_Table/Char_EXCLAMATION_MARK6 ==
  Byte_2 : Constant  Value=c.char_7x7(2, :, c.EXCLAMATION_MARK)  OutDataTypeStr=uint8
  Byte_3 : Constant  Value=c.char_7x7(3, :, c.EXCLAMATION_MARK)  OutDataTypeStr=uint8
  Byte_4 : Constant  Value=c.char_7x7(4, :, c.EXCLAMATION_MARK)  OutDataTypeStr=uint8
  Byte_5 : Constant  Value=c.char_7x7(5, :, c.EXCLAMATION_MARK)  OutDataTypeStr=uint8
  Byte_6 : Constant  Value=c.char_7x7(6, :, c.EXCLAMATION_MARK)  OutDataTypeStr=uint8
  Byte_7 : Constant  Value=c.char_7x7(7, :, c.EXCLAMATION_MARK)  OutDataTypeStr=uint8
  Byte_8 : Constant  Value=c.char_7x7(8, :, c.EXCLAMATION_MARK)  OutDataTypeStr=uint8
  Byte_9 : Constant  Value=c.char_7x7(1, :, c.EXCLAMATION_MARK)  OutDataTypeStr=uint8
  Row_7(1B) : Outport
  Row_6(1B) : Outport  Port=2
  Row_5(1B) : Outport  Port=3
  Row_4(1B) : Outport  Port=4
  Row_3(1B) : Outport  Port=5
  Row_2(1B) : Outport  Port=6
  Row_1(1B) : Outport  Port=7
  Row_0(1B) : Outport  Port=8
  wires:
  Byte_3/1 -> Row_5(1B)/1
  Byte_9/1 -> Row_7(1B)/1
  Byte_7/1 -> Row_1(1B)/1
  Byte_4/1 -> Row_4(1B)/1
  Byte_8/1 -> Row_0(1B)/1
  Byte_2/1 -> Row_6(1B)/1
  Byte_5/1 -> Row_3(1B)/1
  Byte_6/1 -> Row_2(1B)/1

== system pokus07_video/Character_Table/Char_EXCLAMATION_MARK7 ==
  Byte_2 : Constant  Value=c.char_7x7(2, :, c.EXCLAMATION_MARK)  OutDataTypeStr=uint8
  Byte_3 : Constant  Value=c.char_7x7(3, :, c.EXCLAMATION_MARK)  OutDataTypeStr=uint8
  Byte_4 : Constant  Value=c.char_7x7(4, :, c.EXCLAMATION_MARK)  OutDataTypeStr=uint8
  Byte_5 : Constant  Value=c.char_7x7(5, :, c.EXCLAMATION_MARK)  OutDataTypeStr=uint8
  Byte_6 : Constant  Value=c.char_7x7(6, :, c.EXCLAMATION_MARK)  OutDataTypeStr=uint8
  Byte_7 : Constant  Value=c.char_7x7(7, :, c.EXCLAMATION_MARK)  OutDataTypeStr=uint8
  Byte_8 : Constant  Value=c.char_7x7(8, :, c.EXCLAMATION_MARK)  OutDataTypeStr=uint8
  Byte_9 : Constant  Value=c.char_7x7(1, :, c.EXCLAMATION_MARK)  OutDataTypeStr=uint8
  Row_7(1B) : Outport
  Row_6(1B) : Outport  Port=2
  Row_5(1B) : Outport  Port=3
  Row_4(1B) : Outport  Port=4
  Row_3(1B) : Outport  Port=5
  Row_2(1B) : Outport  Port=6
  Row_1(1B) : Outport  Port=7
  Row_0(1B) : Outport  Port=8
  wires:
  Byte_3/1 -> Row_5(1B)/1
  Byte_9/1 -> Row_7(1B)/1
  Byte_7/1 -> Row_1(1B)/1
  Byte_4/1 -> Row_4(1B)/1
  Byte_8/1 -> Row_0(1B)/1
  Byte_2/1 -> Row_6(1B)/1
  Byte_5/1 -> Row_3(1B)/1
  Byte_6/1 -> Row_2(1B)/1

== system pokus07_video/Character_Table/Char_EXCLAMATION_MARK8 ==
  Byte_2 : Constant  Value=c.char_7x7(2, :, c.EXCLAMATION_MARK)  OutDataTypeStr=uint8
  Byte_3 : Constant  Value=c.char_7x7(3, :, c.EXCLAMATION_MARK)  OutDataTypeStr=uint8
  Byte_4 : Constant  Value=c.char_7x7(4, :, c.EXCLAMATION_MARK)  OutDataTypeStr=uint8
  Byte_5 : Constant  Value=c.char_7x7(5, :, c.EXCLAMATION_MARK)  OutDataTypeStr=uint8
  Byte_6 : Constant  Value=c.char_7x7(6, :, c.EXCLAMATION_MARK)  OutDataTypeStr=uint8
  Byte_7 : Constant  Value=c.char_7x7(7, :, c.EXCLAMATION_MARK)  OutDataTypeStr=uint8
  Byte_8 : Constant  Value=c.char_7x7(8, :, c.EXCLAMATION_MARK)  OutDataTypeStr=uint8
  Byte_9 : Constant  Value=c.char_7x7(1, :, c.EXCLAMATION_MARK)  OutDataTypeStr=uint8
  Row_7(1B) : Outport
  Row_6(1B) : Outport  Port=2
  Row_5(1B) : Outport  Port=3
  Row_4(1B) : Outport  Port=4
  Row_3(1B) : Outport  Port=5
  Row_2(1B) : Outport  Port=6
  Row_1(1B) : Outport  Port=7
  Row_0(1B) : Outport  Port=8
  wires:
  Byte_3/1 -> Row_5(1B)/1
  Byte_9/1 -> Row_7(1B)/1
  Byte_7/1 -> Row_1(1B)/1
  Byte_4/1 -> Row_4(1B)/1
  Byte_8/1 -> Row_0(1B)/1
  Byte_2/1 -> Row_6(1B)/1
  Byte_5/1 -> Row_3(1B)/1
  Byte_6/1 -> Row_2(1B)/1

== system pokus07_video/Character_Table/Char_EXCLAMATION_MARK9 ==
  Byte_2 : Constant  Value=c.char_7x7(2, :, c.EXCLAMATION_MARK)  OutDataTypeStr=uint8
  Byte_3 : Constant  Value=c.char_7x7(3, :, c.EXCLAMATION_MARK)  OutDataTypeStr=uint8
  Byte_4 : Constant  Value=c.char_7x7(4, :, c.EXCLAMATION_MARK)  OutDataTypeStr=uint8
  Byte_5 : Constant  Value=c.char_7x7(5, :, c.EXCLAMATION_MARK)  OutDataTypeStr=uint8
  Byte_6 : Constant  Value=c.char_7x7(6, :, c.EXCLAMATION_MARK)  OutDataTypeStr=uint8
  Byte_7 : Constant  Value=c.char_7x7(7, :, c.EXCLAMATION_MARK)  OutDataTypeStr=uint8
  Byte_8 : Constant  Value=c.char_7x7(8, :, c.EXCLAMATION_MARK)  OutDataTypeStr=uint8
  Byte_9 : Constant  Value=c.char_7x7(1, :, c.EXCLAMATION_MARK)  OutDataTypeStr=uint8
  Row_7(1B) : Outport
  Row_6(1B) : Outport  Port=2
  Row_5(1B) : Outport  Port=3
  Row_4(1B) : Outport  Port=4
  Row_3(1B) : Outport  Port=5
  Row_2(1B) : Outport  Port=6
  Row_1(1B) : Outport  Port=7
  Row_0(1B) : Outport  Port=8
  wires:
  Byte_3/1 -> Row_5(1B)/1
  Byte_9/1 -> Row_7(1B)/1
  Byte_7/1 -> Row_1(1B)/1
  Byte_4/1 -> Row_4(1B)/1
  Byte_8/1 -> Row_0(1B)/1
  Byte_2/1 -> Row_6(1B)/1
  Byte_5/1 -> Row_3(1B)/1
  Byte_6/1 -> Row_2(1B)/1

== system pokus07_video/Character_Table/Char_F ==
  Byte_2 : Constant  Value=c.char_7x7(2, :, c.F)  OutDataTypeStr=uint8
  Byte_3 : Constant  Value=c.char_7x7(3, :, c.F)  OutDataTypeStr=uint8
  Byte_4 : Constant  Value=c.char_7x7(4, :, c.F)  OutDataTypeStr=uint8
  Byte_5 : Constant  Value=c.char_7x7(5, :, c.F)  OutDataTypeStr=uint8
  Byte_6 : Constant  Value=c.char_7x7(6, :, c.F)  OutDataTypeStr=uint8
  Byte_7 : Constant  Value=c.char_7x7(7, :, c.F)  OutDataTypeStr=uint8
  Byte_8 : Constant  Value=c.char_7x7(8, :, c.F)  OutDataTypeStr=uint8
  Byte_9 : Constant  Value=c.char_7x7(1, :, c.F)  OutDataTypeStr=uint8
  Row_7(1B) : Outport
  Row_6(1B) : Outport  Port=2
  Row_5(1B) : Outport  Port=3
  Row_4(1B) : Outport  Port=4
  Row_3(1B) : Outport  Port=5
  Row_2(1B) : Outport  Port=6
  Row_1(1B) : Outport  Port=7
  Row_0(1B) : Outport  Port=8
  wires:
  Byte_6/1 -> Row_2(1B)/1
  Byte_8/1 -> Row_0(1B)/1
  Byte_7/1 -> Row_1(1B)/1
  Byte_5/1 -> Row_3(1B)/1
  Byte_9/1 -> Row_7(1B)/1
  Byte_2/1 -> Row_6(1B)/1
  Byte_4/1 -> Row_4(1B)/1
  Byte_3/1 -> Row_5(1B)/1

== system pokus07_video/Character_Table/Char_G ==
  Byte_2 : Constant  Value=c.char_7x7(2, :, c.G)  OutDataTypeStr=uint8
  Byte_3 : Constant  Value=c.char_7x7(3, :, c.G)  OutDataTypeStr=uint8
  Byte_4 : Constant  Value=c.char_7x7(4, :, c.G)  OutDataTypeStr=uint8
  Byte_5 : Constant  Value=c.char_7x7(5, :, c.G)  OutDataTypeStr=uint8
  Byte_6 : Constant  Value=c.char_7x7(6, :, c.G)  OutDataTypeStr=uint8
  Byte_7 : Constant  Value=c.char_7x7(7, :, c.G)  OutDataTypeStr=uint8
  Byte_8 : Constant  Value=c.char_7x7(8, :, c.G)  OutDataTypeStr=uint8
  Byte_9 : Constant  Value=c.char_7x7(1, :, c.G)  OutDataTypeStr=uint8
  Row_7(1B) : Outport
  Row_6(1B) : Outport  Port=2
  Row_5(1B) : Outport  Port=3
  Row_4(1B) : Outport  Port=4
  Row_3(1B) : Outport  Port=5
  Row_2(1B) : Outport  Port=6
  Row_1(1B) : Outport  Port=7
  Row_0(1B) : Outport  Port=8
  wires:
  Byte_2/1 -> Row_6(1B)/1
  Byte_3/1 -> Row_5(1B)/1
  Byte_9/1 -> Row_7(1B)/1
  Byte_4/1 -> Row_4(1B)/1
  Byte_8/1 -> Row_0(1B)/1
  Byte_6/1 -> Row_2(1B)/1
  Byte_7/1 -> Row_1(1B)/1
  Byte_5/1 -> Row_3(1B)/1

== system pokus07_video/Character_Table/Char_GREATER_THAN ==
  Byte_2 : Constant  Value=c.char_7x7(2, :, c.GREATER_THAN)  OutDataTypeStr=uint8
  Byte_3 : Constant  Value=c.char_7x7(3, :, c.GREATER_THAN)  OutDataTypeStr=uint8
  Byte_4 : Constant  Value=c.char_7x7(4, :, c.GREATER_THAN)  OutDataTypeStr=uint8
  Byte_5 : Constant  Value=c.char_7x7(5, :, c.GREATER_THAN)  OutDataTypeStr=uint8
  Byte_6 : Constant  Value=c.char_7x7(6, :, c.GREATER_THAN)  OutDataTypeStr=uint8
  Byte_7 : Constant  Value=c.char_7x7(7, :, c.GREATER_THAN)  OutDataTypeStr=uint8
  Byte_8 : Constant  Value=c.char_7x7(8, :, c.GREATER_THAN)  OutDataTypeStr=uint8
  Byte_9 : Constant  Value=c.char_7x7(1, :, c.GREATER_THAN)  OutDataTypeStr=uint8
  Row_7(1B) : Outport
  Row_6(1B) : Outport  Port=2
  Row_5(1B) : Outport  Port=3
  Row_4(1B) : Outport  Port=4
  Row_3(1B) : Outport  Port=5
  Row_2(1B) : Outport  Port=6
  Row_1(1B) : Outport  Port=7
  Row_0(1B) : Outport  Port=8
  wires:
  Byte_3/1 -> Row_5(1B)/1
  Byte_9/1 -> Row_7(1B)/1
  Byte_7/1 -> Row_1(1B)/1
  Byte_4/1 -> Row_4(1B)/1
  Byte_8/1 -> Row_0(1B)/1
  Byte_2/1 -> Row_6(1B)/1
  Byte_5/1 -> Row_3(1B)/1
  Byte_6/1 -> Row_2(1B)/1

== system pokus07_video/Character_Table/Char_H ==
  Byte_2 : Constant  Value=c.char_7x7(2, :, c.H)  OutDataTypeStr=uint8
  Byte_3 : Constant  Value=c.char_7x7(3, :, c.H)  OutDataTypeStr=uint8
  Byte_4 : Constant  Value=c.char_7x7(4, :, c.H)  OutDataTypeStr=uint8
  Byte_5 : Constant  Value=c.char_7x7(5, :, c.H)  OutDataTypeStr=uint8
  Byte_6 : Constant  Value=c.char_7x7(6, :, c.H)  OutDataTypeStr=uint8
  Byte_7 : Constant  Value=c.char_7x7(7, :, c.H)  OutDataTypeStr=uint8
  Byte_8 : Constant  Value=c.char_7x7(8, :, c.H)  OutDataTypeStr=uint8
  Byte_9 : Constant  Value=c.char_7x7(1, :, c.H)  OutDataTypeStr=uint8
  Row_7(1B) : Outport
  Row_6(1B) : Outport  Port=2
  Row_5(1B) : Outport  Port=3
  Row_4(1B) : Outport  Port=4
  Row_3(1B) : Outport  Port=5
  Row_2(1B) : Outport  Port=6
  Row_1(1B) : Outport  Port=7
  Row_0(1B) : Outport  Port=8
  wires:
  Byte_9/1 -> Row_7(1B)/1
  Byte_4/1 -> Row_4(1B)/1
  Byte_6/1 -> Row_2(1B)/1
  Byte_7/1 -> Row_1(1B)/1
  Byte_5/1 -> Row_3(1B)/1
  Byte_8/1 -> Row_0(1B)/1
  Byte_2/1 -> Row_6(1B)/1
  Byte_3/1 -> Row_5(1B)/1

== system pokus07_video/Character_Table/Char_I ==
  Byte_2 : Constant  Value=c.char_7x7(2, :, c.I)  OutDataTypeStr=uint8
  Byte_3 : Constant  Value=c.char_7x7(3, :, c.I)  OutDataTypeStr=uint8
  Byte_4 : Constant  Value=c.char_7x7(4, :, c.I)  OutDataTypeStr=uint8
  Byte_5 : Constant  Value=c.char_7x7(5, :, c.I)  OutDataTypeStr=uint8
  Byte_6 : Constant  Value=c.char_7x7(6, :, c.I)  OutDataTypeStr=uint8
  Byte_7 : Constant  Value=c.char_7x7(7, :, c.I)  OutDataTypeStr=uint8
  Byte_8 : Constant  Value=c.char_7x7(8, :, c.I)  OutDataTypeStr=uint8
  Byte_9 : Constant  Value=c.char_7x7(1, :, c.I)  OutDataTypeStr=uint8
  Row_7(1B) : Outport
  Row_6(1B) : Outport  Port=2
  Row_5(1B) : Outport  Port=3
  Row_4(1B) : Outport  Port=4
  Row_3(1B) : Outport  Port=5
  Row_2(1B) : Outport  Port=6
  Row_1(1B) : Outport  Port=7
  Row_0(1B) : Outport  Port=8
  wires:
  Byte_2/1 -> Row_6(1B)/1
  Byte_3/1 -> Row_5(1B)/1
  Byte_5/1 -> Row_3(1B)/1
  Byte_7/1 -> Row_1(1B)/1
  Byte_9/1 -> Row_7(1B)/1
  Byte_4/1 -> Row_4(1B)/1
  Byte_8/1 -> Row_0(1B)/1
  Byte_6/1 -> Row_2(1B)/1

== system pokus07_video/Character_Table/Char_J ==
  Byte_2 : Constant  Value=c.char_7x7(2, :, c.J)  OutDataTypeStr=uint8
  Byte_3 : Constant  Value=c.char_7x7(3, :, c.J)  OutDataTypeStr=uint8
  Byte_4 : Constant  Value=c.char_7x7(4, :, c.J)  OutDataTypeStr=uint8
  Byte_5 : Constant  Value=c.char_7x7(5, :, c.J)  OutDataTypeStr=uint8
  Byte_6 : Constant  Value=c.char_7x7(6, :, c.J)  OutDataTypeStr=uint8
  Byte_7 : Constant  Value=c.char_7x7(7, :, c.J)  OutDataTypeStr=uint8
  Byte_8 : Constant  Value=c.char_7x7(8, :, c.J)  OutDataTypeStr=uint8
  Byte_9 : Constant  Value=c.char_7x7(1, :, c.J)  OutDataTypeStr=uint8
  Row_7(1B) : Outport
  Row_6(1B) : Outport  Port=2
  Row_5(1B) : Outport  Port=3
  Row_4(1B) : Outport  Port=4
  Row_3(1B) : Outport  Port=5
  Row_2(1B) : Outport  Port=6
  Row_1(1B) : Outport  Port=7
  Row_0(1B) : Outport  Port=8
  wires:
  Byte_8/1 -> Row_0(1B)/1
  Byte_9/1 -> Row_7(1B)/1
  Byte_4/1 -> Row_4(1B)/1
  Byte_6/1 -> Row_2(1B)/1
  Byte_7/1 -> Row_1(1B)/1
  Byte_5/1 -> Row_3(1B)/1
  Byte_2/1 -> Row_6(1B)/1
  Byte_3/1 -> Row_5(1B)/1

== system pokus07_video/Character_Table/Char_K ==
  Byte_2 : Constant  Value=c.char_7x7(2, :, c.K)  OutDataTypeStr=uint8
  Byte_3 : Constant  Value=c.char_7x7(3, :, c.K)  OutDataTypeStr=uint8
  Byte_4 : Constant  Value=c.char_7x7(4, :, c.K)  OutDataTypeStr=uint8
  Byte_5 : Constant  Value=c.char_7x7(5, :, c.K)  OutDataTypeStr=uint8
  Byte_6 : Constant  Value=c.char_7x7(6, :, c.K)  OutDataTypeStr=uint8
  Byte_7 : Constant  Value=c.char_7x7(7, :, c.K)  OutDataTypeStr=uint8
  Byte_8 : Constant  Value=c.char_7x7(8, :, c.K)  OutDataTypeStr=uint8
  Byte_9 : Constant  Value=c.char_7x7(1, :, c.K)  OutDataTypeStr=uint8
  Row_7(1B) : Outport
  Row_6(1B) : Outport  Port=2
  Row_5(1B) : Outport  Port=3
  Row_4(1B) : Outport  Port=4
  Row_3(1B) : Outport  Port=5
  Row_2(1B) : Outport  Port=6
  Row_1(1B) : Outport  Port=7
  Row_0(1B) : Outport  Port=8
  wires:
  Byte_4/1 -> Row_4(1B)/1
  Byte_8/1 -> Row_0(1B)/1
  Byte_7/1 -> Row_1(1B)/1
  Byte_2/1 -> Row_6(1B)/1
  Byte_9/1 -> Row_7(1B)/1
  Byte_5/1 -> Row_3(1B)/1
  Byte_3/1 -> Row_5(1B)/1
  Byte_6/1 -> Row_2(1B)/1

== system pokus07_video/Character_Table/Char_L ==
  Byte_2 : Constant  Value=c.char_7x7(2, :, c.L)  OutDataTypeStr=uint8
  Byte_3 : Constant  Value=c.char_7x7(3, :, c.L)  OutDataTypeStr=uint8
  Byte_4 : Constant  Value=c.char_7x7(4, :, c.L)  OutDataTypeStr=uint8
  Byte_5 : Constant  Value=c.char_7x7(5, :, c.L)  OutDataTypeStr=uint8
  Byte_6 : Constant  Value=c.char_7x7(6, :, c.L)  OutDataTypeStr=uint8
  Byte_7 : Constant  Value=c.char_7x7(7, :, c.L)  OutDataTypeStr=uint8
  Byte_8 : Constant  Value=c.char_7x7(8, :, c.L)  OutDataTypeStr=uint8
  Byte_9 : Constant  Value=c.char_7x7(1, :, c.L)  OutDataTypeStr=uint8
  Row_7(1B) : Outport
  Row_6(1B) : Outport  Port=2
  Row_5(1B) : Outport  Port=3
  Row_4(1B) : Outport  Port=4
  Row_3(1B) : Outport  Port=5
  Row_2(1B) : Outport  Port=6
  Row_1(1B) : Outport  Port=7
  Row_0(1B) : Outport  Port=8
  wires:
  Byte_8/1 -> Row_0(1B)/1
  Byte_5/1 -> Row_3(1B)/1
  Byte_3/1 -> Row_5(1B)/1
  Byte_9/1 -> Row_7(1B)/1
  Byte_4/1 -> Row_4(1B)/1
  Byte_7/1 -> Row_1(1B)/1
  Byte_6/1 -> Row_2(1B)/1
  Byte_2/1 -> Row_6(1B)/1

== system pokus07_video/Character_Table/Char_LESS_THAN ==
  Byte_2 : Constant  Value=c.char_7x7(2, :, c.LESS_THAN)  OutDataTypeStr=uint8
  Byte_3 : Constant  Value=c.char_7x7(3, :, c.LESS_THAN)  OutDataTypeStr=uint8
  Byte_4 : Constant  Value=c.char_7x7(4, :, c.LESS_THAN)  OutDataTypeStr=uint8
  Byte_5 : Constant  Value=c.char_7x7(5, :, c.LESS_THAN)  OutDataTypeStr=uint8
  Byte_6 : Constant  Value=c.char_7x7(6, :, c.LESS_THAN)  OutDataTypeStr=uint8
  Byte_7 : Constant  Value=c.char_7x7(7, :, c.LESS_THAN)  OutDataTypeStr=uint8
  Byte_8 : Constant  Value=c.char_7x7(8, :, c.LESS_THAN)  OutDataTypeStr=uint8
  Byte_9 : Constant  Value=c.char_7x7(1, :, c.LESS_THAN)  OutDataTypeStr=uint8
  Row_7(1B) : Outport
  Row_6(1B) : Outport  Port=2
  Row_5(1B) : Outport  Port=3
  Row_4(1B) : Outport  Port=4
  Row_3(1B) : Outport  Port=5
  Row_2(1B) : Outport  Port=6
  Row_1(1B) : Outport  Port=7
  Row_0(1B) : Outport  Port=8
  wires:
  Byte_3/1 -> Row_5(1B)/1
  Byte_9/1 -> Row_7(1B)/1
  Byte_7/1 -> Row_1(1B)/1
  Byte_4/1 -> Row_4(1B)/1
  Byte_8/1 -> Row_0(1B)/1
  Byte_2/1 -> Row_6(1B)/1
  Byte_5/1 -> Row_3(1B)/1
  Byte_6/1 -> Row_2(1B)/1

== system pokus07_video/Character_Table/Char_M ==
  Byte_2 : Constant  Value=c.char_7x7(2, :, c.M)  OutDataTypeStr=uint8
  Byte_3 : Constant  Value=c.char_7x7(3, :, c.M)  OutDataTypeStr=uint8
  Byte_4 : Constant  Value=c.char_7x7(4, :, c.M)  OutDataTypeStr=uint8
  Byte_5 : Constant  Value=c.char_7x7(5, :, c.M)  OutDataTypeStr=uint8
  Byte_6 : Constant  Value=c.char_7x7(6, :, c.M)  OutDataTypeStr=uint8
  Byte_7 : Constant  Value=c.char_7x7(7, :, c.M)  OutDataTypeStr=uint8
  Byte_8 : Constant  Value=c.char_7x7(8, :, c.M)  OutDataTypeStr=uint8
  Byte_9 : Constant  Value=c.char_7x7(1, :, c.M)  OutDataTypeStr=uint8
  Row_7(1B) : Outport
  Row_6(1B) : Outport  Port=2
  Row_5(1B) : Outport  Port=3
  Row_4(1B) : Outport  Port=4
  Row_3(1B) : Outport  Port=5
  Row_2(1B) : Outport  Port=6
  Row_1(1B) : Outport  Port=7
  Row_0(1B) : Outport  Port=8
  wires:
  Byte_3/1 -> Row_5(1B)/1
  Byte_9/1 -> Row_7(1B)/1
  Byte_7/1 -> Row_1(1B)/1
  Byte_4/1 -> Row_4(1B)/1
  Byte_8/1 -> Row_0(1B)/1
  Byte_2/1 -> Row_6(1B)/1
  Byte_5/1 -> Row_3(1B)/1
  Byte_6/1 -> Row_2(1B)/1

== system pokus07_video/Character_Table/Char_MINUS ==
  Byte_2 : Constant  Value=c.char_7x7(2, :, c.MINUS)  OutDataTypeStr=uint8
  Byte_3 : Constant  Value=c.char_7x7(3, :, c.MINUS)  OutDataTypeStr=uint8
  Byte_4 : Constant  Value=c.char_7x7(4, :, c.MINUS)  OutDataTypeStr=uint8
  Byte_5 : Constant  Value=c.char_7x7(5, :, c.MINUS)  OutDataTypeStr=uint8
  Byte_6 : Constant  Value=c.char_7x7(6, :, c.MINUS)  OutDataTypeStr=uint8
  Byte_7 : Constant  Value=c.char_7x7(7, :, c.MINUS)  OutDataTypeStr=uint8
  Byte_8 : Constant  Value=c.char_7x7(8, :, c.MINUS)  OutDataTypeStr=uint8
  Byte_9 : Constant  Value=c.char_7x7(1, :, c.MINUS)  OutDataTypeStr=uint8
  Row_7(1B) : Outport
  Row_6(1B) : Outport  Port=2
  Row_5(1B) : Outport  Port=3
  Row_4(1B) : Outport  Port=4
  Row_3(1B) : Outport  Port=5
  Row_2(1B) : Outport  Port=6
  Row_1(1B) : Outport  Port=7
  Row_0(1B) : Outport  Port=8
  wires:
  Byte_3/1 -> Row_5(1B)/1
  Byte_9/1 -> Row_7(1B)/1
  Byte_7/1 -> Row_1(1B)/1
  Byte_4/1 -> Row_4(1B)/1
  Byte_8/1 -> Row_0(1B)/1
  Byte_2/1 -> Row_6(1B)/1
  Byte_5/1 -> Row_3(1B)/1
  Byte_6/1 -> Row_2(1B)/1
